simulink model "Gesamtsystem_Prototyp25_01_3"  (R2021b)
settings: Solver=FixedStepDiscrete  StartTime=0.0  StopTime=Inf  RelTol=1e-3  EnableMultiTasking=on
undefined symbols (not defined in the file): Down, GPTRIP1SEL, GPTRIP2SEL, magnitude, TZ1, TZ2, Up
libraries: c2837xDlib x18, hdlsllib x10, simulink x5, c2802xlib x5, c280xlib x3, dspsigops x3, commsequence2 x2, idelinklib_common x2, mcbcontrolslib x2, c2000lib x1, dspstat3 x1
(part 1 of 3)
settings Model: SimulationMode=external  ExtModeTrigDuration=8  Creator=The MathWorks, Inc.  LastModifiedBy=richa
settings SolverCC: AlgebraicLoopSolver=TrustRegion
settings OptimizationCC: DefaultUnderspecifiedDataType=single  EnhancedBackFolding=on  PassReuseOutputArgsAs=Individual arguments  MaxStackSize=1024  OptimizeBlockOrder=speed  DifferentSizesBufferReuse=on  OptimizationCustomize=off  DenormalBehavior=FlushToZero  EfficientTunableParamExpr=on
settings DebuggingCC: MultiTaskRateTransMsg=warning  ParameterTunabilityLossMsg=error  SFMachineParentedDataDiag=warning
settings HardwareCC: ProdBitPerChar=16  ProdBitPerInt=16  ProdBitPerPointer=32  ProdBitPerSizeT=32  ProdBitPerPtrDiffT=32  ProdLargestAtomicInteger=Integer  ProdLargestAtomicFloat=None  ProdWordSize=16  ProdLongLongMode=on  ProdHWDeviceType=Texas Instruments->C2000
settings SFSimCC: SimCustomSourceCode="#include \"i2c_reset.c\""  SimCustomHeaderCode="#include \"i2c_reset.h\""  MATLABDynamicMemAlloc=off
settings RTWCC: Description=Embedded Coder  SystemTargetFile=ert.tlc  HardwareBoard=TI Delfino F28379D LaunchPad  TemplateMakefile=ert_default_tmf  GenerateReport=on  RTWUseSimCustomCode=on  CustomSourceCode="#include \"i2c_reset.c\""  CustomHeaderCode="#include \"i2c_reset.h\""  Toolchain=Texas Instruments Code Composer Studio (C2000)
settings CodeAppCC: ForceParamTrailComments=on  IgnoreCustomStorageClasses=off  OperatorAnnotations=on  SimulinkDataObjDesc=on  SFDataObjDesc=on  InsertBlockDesc=on
settings ERTTargetCC: CodeReplacementLibrary=TI C28x  SupportContinuousTime=on  ExtMode=on  ExtModeTransport=4  ExtModeStaticAlloc=on  ExtModeStaticAllocSize=10000  ExtModeMexFile=ext_xcp  ExtModeMexArgs=1 7 5000000  ExtModeIntrfLevel=Level2 - Open

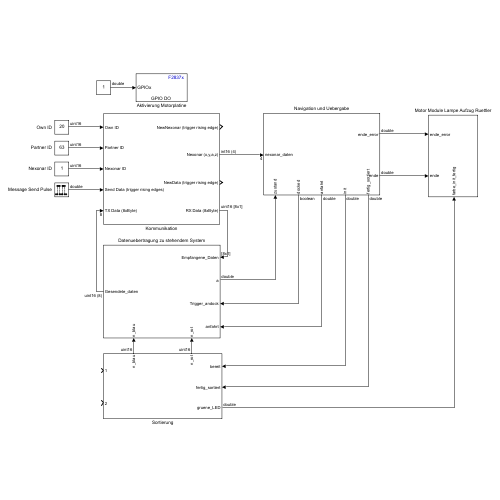
[thumbnail: Simulink's stored preview of the top-level diagram]
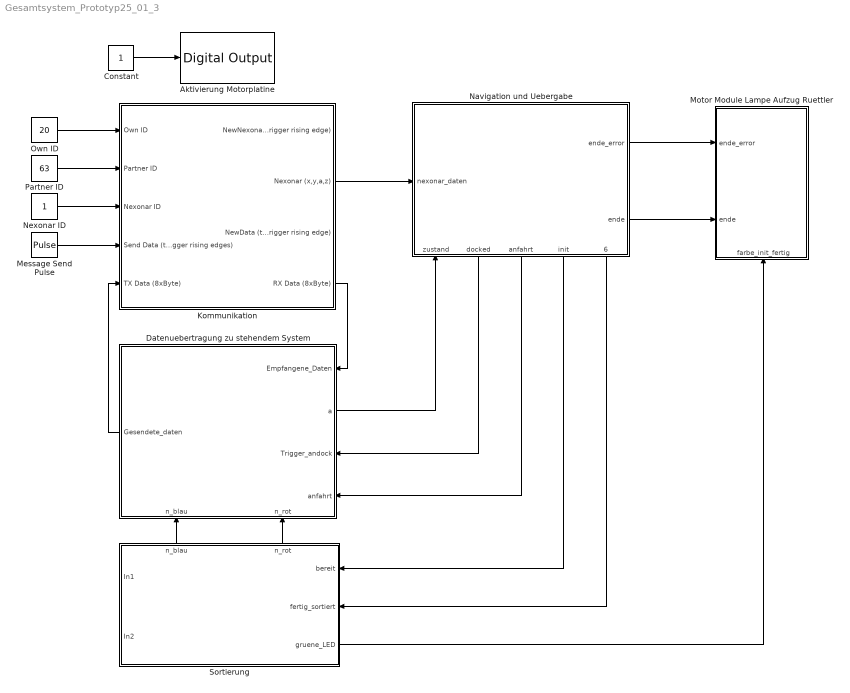
== system Gesamtsystem_Prototyp25_01_3 ==
  Aktivierung Motorplatine : c2837xDlib/Digital Output  GPIO_Number=GPIO48~GPIO55  GPIO_Bit0=off  GPIO_BIT0_Toggle=on  GPIO_Bit1=off  GPIO_BIT1_Toggle=off  GPIO_Bit2=off  GPIO_BIT2_Toggle=off  GPIO_Bit3=off  GPIO_BIT3_Toggle=off  GPIO_Bit4=on  GPIO_BIT4_Toggle=on  GPIO_Bit5=off  GPIO_BIT5_Toggle=off  GPIO_Bit6=off  GPIO_BIT6_Toggle=off  GPIO_Bit7=off  GPIO_BIT7_Toggle=off
      settings: SourceProductBaseCode=TIC2000
  Constant : Constant
  Datenuebertragung zu stehendem System : Subsystem
      settings: PortSchema="{\"entries\":[{\"content\":{\"sides\":[{\"content\":{\"connectorIds\":[\"Out2\"]},\"type\":\"ConnectorPlacement.EquallySpacedRectSide\",\"uuid\":\"280a4ad7-2b89-47a7-b582-5b9e1aa8e579\"},{\"content\":{\"connectorIds\":[\"In3\",\"Out1\",\"In4\",\"In5\"],\"side\":\"RIGHT\"},\"type\":\"ConnectorPlacement.EquallySpacedRectSide\",\"uuid\":\"026a8d37-e820-494f-976a-b1ab356a46bf\"},{\"content\":{\"connectorIds\":[],\"side\":\"TOP\"},\"type\":\"ConnectorPlacement.EquallySpacedRectSide\",\"uuid\":\"c41355c1-e8ef-4a5b-90ea-c5b98acbcd23\"},{\"content\":{\"connectorIds\":[\"In1\",\"In2\"],\"side\":\"BOTTOM\"},\"type\":\"ConnectorPlacement.EquallySpacedRectSide\",\"uuid\":\"0f189695-a2e5-45de-b8d0-0b48a4f2d2d4\"}]},\"type\":\"ConnectorPlacement.EquallySpacedConnector\",\"uuid\":\"44cb629b-e0dd-4ad8-b455-e727a6a25bea\"}],\"packageUris\":[\"http://schema.mathworks.com/mf0/Connector/R2020b\"],\"version\":\"1.0\"}"
  Kommunikation : Subsystem
  Message Send Pulse : DiscretePulseGenerator  SampleTime=0.25
  Motor Module Lampe Aufzug Ruettler : Subsystem
      settings: PortSchema="{\"entries\":[{\"content\":{\"sides\":[{\"content\":{\"connectorIds\":[\"In1\",\"In2\"]},\"type\":\"ConnectorPlacement.EquallySpacedRectSide\",\"uuid\":\"9123dc57-6e13-4d06-96d5-694d4c57ade7\"},{\"content\":{\"connectorIds\":[],\"side\":\"RIGHT\"},\"type\":\"ConnectorPlacement.EquallySpacedRectSide\",\"uuid\":\"65464e42-9400-426f-8ced-3069c16bd5e7\"},{\"content\":{\"connectorIds\":[],\"side\":\"TOP\"},\"type\":\"ConnectorPlacement.EquallySpacedRectSide\",\"uuid\":\"b48c1543-2088-461c-846d-d08a40b96f4c\"},{\"content\":{\"connectorIds\":[\"In3\"],\"side\":\"BOTTOM\"},\"type\":\"ConnectorPlacement.EquallySpacedRectSide\",\"uuid\":\"aa8ff81a-6422-494d-aeab-2069a4a6b426\"}]},\"type\":\"ConnectorPlacement.EquallySpacedConnector\",\"uuid\":\"98b07be5-fb16-44db-b7cc-951c09166bfd\"}],\"packageUris\":[\"http://schema.mathworks.com/mf0/Connector/R2020b\"],\"version\":\"1.0\"}"
  Navigation und Uebergabe : Subsystem
      settings: PortSchema="{\"entries\":[{\"content\":{\"sides\":[{\"content\":{\"connectorIds\":[\"In1\"]},\"type\":\"ConnectorPlacement.EquallySpacedRectSide\",\"uuid\":\"dfc964e5-dd2b-4b2e-9c3a-c7814fa8e123\"},{\"content\":{\"connectorIds\":[\"Out1\",\"Out2\"],\"side\":\"RIGHT\"},\"type\":\"ConnectorPlacement.EquallySpacedRectSide\",\"uuid\":\"39fc11e7-81f7-4c6b-bd33-df7afb59ff58\"},{\"content\":{\"connectorIds\":[],\"side\":\"TOP\"},\"type\":\"ConnectorPlacement.EquallySpacedRectSide\",\"uuid\":\"36c4a621-1407-48e7-9ea9-d5e57de15753\"},{\"content\":{\"connectorIds\":[\"In2\",\"Out3\",\"Out4\",\"Out5\",\"Out6\"],\"side\":\"BOTTOM\"},\"type\":\"ConnectorPlacement.EquallySpacedRectSide\",\"uuid\":\"43cd8641-88b7-45a0-ae78-0764539c8380\"}]},\"type\":\"ConnectorPlacement.EquallySpacedConnector\",\"uuid\":\"ac412e3d-8275-4bb9-9e3f-1b0a94176768\"}],\"packageUris\":[\"http://schema.mathworks.com/mf0/Connector/R2020b\"],\"version\":\"1.0\"}"
  Nexonar ID : Constant  OutDataTypeStr=uint16
  Own ID : Constant  Value=20  OutDataTypeStr=uint16
  Partner ID : Constant  Value=63  OutDataTypeStr=uint16
  Sortierung : Subsystem
      settings: PortSchema="{\"entries\":[{\"content\":{\"sides\":[{\"content\":{\"connectorIds\":[\"In1\",\"In2\"]},\"type\":\"ConnectorPlacement.EquallySpacedRectSide\",\"uuid\":\"ab30f80d-c1d3-46e0-874b-ff067c3feed5\"},{\"content\":{\"connectorIds\":[\"In3\",\"In4\",\"Out1\"],\"side\":\"RIGHT\"},\"type\":\"ConnectorPlacement.EquallySpacedRectSide\",\"uuid\":\"516d9c97-20f8-430b-a7d3-5b8718eca889\"},{\"content\":{\"connectorIds\":[\"Out2\",\"Out3\"],\"side\":\"TOP\"},\"type\":\"ConnectorPlacement.EquallySpacedRectSide\",\"uuid\":\"26f872a1-b740-4d7b-a87d-ca1faf51abaa\"},{\"content\":{\"connectorIds\":[],\"side\":\"BOTTOM\"},\"type\":\"ConnectorPlacement.EquallySpacedRectSide\",\"uuid\":\"97241500-f762-4060-9f54-e0d97a9e1284\"}]},\"type\":\"ConnectorPlacement.EquallySpacedConnector\",\"uuid\":\"cf514a40-a14e-4820-a098-62891cb48e81\"}],\"packageUris\":[\"http://schema.mathworks.com/mf0/Connector/R2020b\"],\"version\":\"1.0\"}"
  wires:
  Constant/1 -> Aktivierung Motorplatine/1
  Partner ID/1 -> Kommunikation/2(Partner ID)
  Own ID/1 -> Kommunikation/1(Own ID)
  Nexonar ID/1 -> Kommunikation/3(Nexonar ID)
  Message Send Pulse/1 -> Kommunikation/4(Send Data (trigger rising edges))
  Kommunikation/2(Nexonar (x,y,a,z)) -> Navigation und Uebergabe/1(nexonar_daten)
  Navigation und Uebergabe/2(ende) -> Motor Module Lampe Aufzug Ruettler/2(ende)
  Kommunikation/4(RX Data (8xByte)) -> Datenuebertragung zu stehendem System/3(Empfangene_Daten)
  Datenuebertragung zu stehendem System/2(Gesendete_daten) -> Kommunikation/5(TX Data (8xByte))
  Datenuebertragung zu stehendem System/1(a) -> Navigation und Uebergabe/2(zustand)
  Sortierung/2(n_blau) -> Datenuebertragung zu stehendem System/1(n_blau)
  Sortierung/3(n_rot) -> Datenuebertragung zu stehendem System/2(n_rot)
  Navigation und Uebergabe/4(anfahrt) -> Datenuebertragung zu stehendem System/5(anfahrt)
  Navigation und Uebergabe/5(init) -> Sortierung/3(bereit)
  Sortierung/1(gruene_LED) -> Motor Module Lampe Aufzug Ruettler/3(farbe_init_fertig)
  Navigation und Uebergabe/3(docked) -> Datenuebertragung zu stehendem System/4(Trigger_andock)
  Navigation und Uebergabe/1(ende_error) -> Motor Module Lampe Aufzug Ruettler/1(ende_error)
  Navigation und Uebergabe/6(fertig_sortiert) -> Sortierung/4(fertig_sortiert)

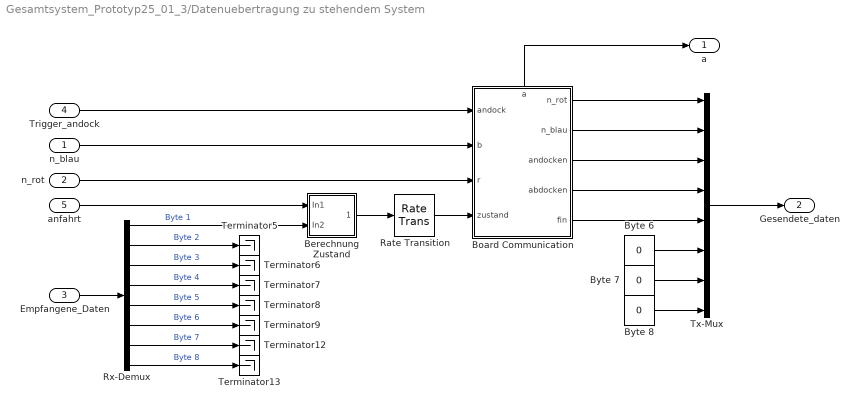
== system Gesamtsystem_Prototyp25_01_3/Datenuebertragung zu stehendem System ==
  n_blau : Inport
  n_rot : Inport  Port=2
  Empfangene_Daten : Inport  Port=3
  Trigger_andock : Inport  Port=4
  anfahrt : Inport  Port=5
  Berechnung Zustand : Subsystem
  Board Communication : Stateflow chart  TreatAsAtomicUnit=on
      settings: PortSchema="{\"entries\":[{\"content\":{\"sides\":[{\"content\":{\"connectorIds\":[\"In4\",\"In1\",\"In2\",\"In3\"]},\"type\":\"ConnectorPlacement.EquallySpacedRectSide\",\"uuid\":\"faa8cb3d-0fdf-435a-9df5-bd02dffb58bc\"},{\"content\":{\"connectorIds\":[\"Out1\",\"Out5\",\"Out3\",\"Out4\",\"Out6\"],\"side\":\"RIGHT\"},\"type\":\"ConnectorPlacement.EquallySpacedRectSide\",\"uuid\":\"4764847e-6149-4239-b002-0e5a6e767122\"},{\"content\":{\"connectorIds\":[\"Out2\"],\"side\":\"TOP\"},\"type\":\"ConnectorPlacement.EquallySpacedRectSide\",\"uuid\":\"2cc71a59-6d23-41ec-a2d6-96294ff626b2\"}]},\"type\":\"ConnectorPlacement.EquallySpacedConnector\",\"uuid\":\"aa42c799-a033-4d4d-b66c-54ab2872aaa8\"}],\"packageUris\":[\"http://schema.mathworks.com/mf0/Connector/R2020b\"],\"version\":\"1.0\"}"
  Byte 6 : Constant  Value=0  OutDataTypeStr=uint16
  Byte 7 : Constant  Value=0  OutDataTypeStr=uint16
  Byte 8 : Constant  Value=0  OutDataTypeStr=uint16
  Rate Transition : RateTransition  OutPortSampleTime=0.2
  Rx-Demux : Demux  Outputs=8
  Terminator{5..9,12..13} (7 alike) : Terminator
  Tx-Mux : Mux  Inputs=8
  a : Outport
  Gesendete_daten : Outport  Port=2
  wires:
  Rx-Demux/3 -> Terminator6/1  "Byte 3"
  Board Communication/3(andocken) -> Tx-Mux/3
  Rx-Demux/1 -> Berechnung Zustand/2(In2)  "Byte 1"
  Rx-Demux/6 -> Terminator9/1  "Byte 6"
  Berechnung Zustand/1(zustand) -> Rate Transition/1
  Board Communication/5(n_blau) -> Tx-Mux/2
  Rx-Demux/4 -> Terminator7/1  "Byte 4"
  Byte 8/1 -> Tx-Mux/8
  Byte 7/1 -> Tx-Mux/7
  Rx-Demux/5 -> Terminator8/1  "Byte 5"
  Rx-Demux/8 -> Terminator13/1  "Byte 8"
  Byte 6/1 -> Tx-Mux/6
  Rx-Demux/7 -> Terminator12/1  "Byte 7"
  Board Communication/6(fin) -> Tx-Mux/5
  Tx-Mux/1 -> Gesendete_daten/1
  Board Communication/4(abdocken) -> Tx-Mux/4
  Rx-Demux/2 -> Terminator5/1  "Byte 2"
  Board Communication/1(n_rot) -> Tx-Mux/1
  Empfangene_Daten/1 -> Rx-Demux/1
  n_rot/1 -> Board Communication/2(r)
  Trigger_andock/1 -> Board Communication/4(andock)
  n_blau/1 -> Board Communication/1(b)
  Board Communication/2(a) -> a/1
  Rate Transition/1 -> Board Communication/3(zustand)
  anfahrt/1 -> Berechnung Zustand/1(In1)

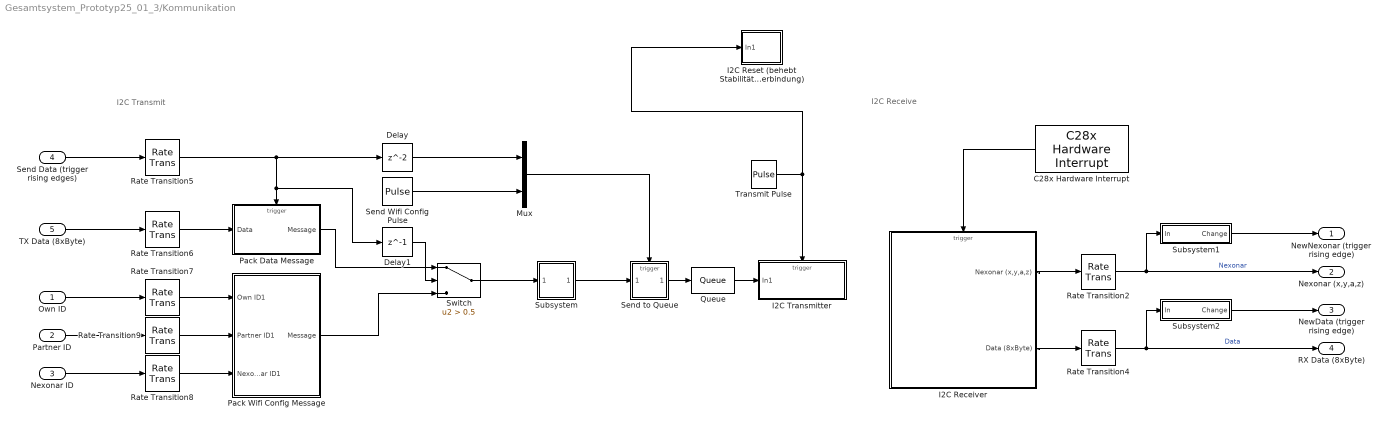
== system Gesamtsystem_Prototyp25_01_3/Kommunikation ==
  note: I2C Receive
  note: I2C Transmit
  Own ID : Inport
  Partner ID : Inport  Port=2
  Nexonar ID : Inport  Port=3
  Send Data (trigger rising edges) : Inport  Port=4
  TX Data (8xByte) : Inport  Port=5
  C28x Hardware Interrupt : c2000lib/Scheduling/C28x Hardware Interrupt  irqnumbers=8  pienumbers=2  irqpriorities=30  irqpreempts=0  showinput=off  dspchiptype=C280X
      settings: SourceProductBaseCode=TIC2000
  Delay : Delay
  Delay1 : Delay  DelayLength=1
  I2C Receiver : Subsystem  TreatAsAtomicUnit=on
  I2C Reset (behebt Stabilitätsprobleme der I2C-Verbindung) : Subsystem
  I2C Transmitter : Subsystem
  Mux : Mux  Inputs=2
  Pack Data Message : Subsystem
  Pack Wifi Config Message : Subsystem
  Queue : Queue  InputPortMessageModes=m  OutputPortMessageModes=m  OverwriteOldest=on  Capacity=16
  Rate Transition2 : RateTransition  Deterministic=off  OutPortSampleTime=0.01
  Rate Transition4 : RateTransition  Deterministic=off  OutPortSampleTime=0.01
  Rate Transition{5..9} (5 alike) : RateTransition  Deterministic=off  OutPortSampleTimeOpt=Inherit  OutPortSampleTime=0.01
  Send Wifi Config Pulse : DiscretePulseGenerator  Period=10  PhaseDelay=30  SampleTime=0.01
  Send to Queue : Subsystem
  Subsystem : Subsystem
  Subsystem1 : Subsystem
  Subsystem2 : Subsystem
  Switch : Switch  Criteria=u2 > Threshold  Threshold=0.5
  Transmit Pulse : DiscretePulseGenerator  Period=100  PulseWidth=5  SampleTime=0.001
  NewNexonar (trigger rising edge) : Outport
  Nexonar (x,y,a,z) : Outport  Port=2
  NewData (trigger rising edge) : Outport  Port=3
  RX Data (8xByte) : Outport  Port=4
  wires:
  I2C Receiver/1(Nexonar (x,y,a,z)) -> Rate Transition2/1
  Rate Transition2/1 -> Subsystem1/1(In), Nexonar (x,y,a,z)/1  "Nexonar"
  C28x Hardware Interrupt/1 -> I2C Receiver/Trigger
  I2C Receiver/2(Data (8xByte)) -> Rate Transition4/1
  Rate Transition4/1 -> Subsystem2/1(In), RX Data (8xByte)/1  "Data"
  Queue/1 -> I2C Transmitter/1(In1)
  Send to Queue/1(Out1) -> Queue/1
  Pack Data Message/1(Message) -> Switch/1
  Pack Wifi Config Message/1(Message) -> Switch/3
  Delay/1 -> Mux/1
  Mux/1 -> Send to Queue/Trigger
  Delay1/1 -> Switch/2
  Send Data (trigger rising edges)/1 -> Rate Transition5/1
  TX Data (8xByte)/1 -> Rate Transition6/1
  Rate Transition6/1 -> Pack Data Message/1(Data)
  Rate Transition9/1 -> Pack Wifi Config Message/2(Partner ID1)
  Partner ID/1 -> Rate Transition9/1
  Own ID/1 -> Rate Transition7/1
  Rate Transition7/1 -> Pack Wifi Config Message/1(Own ID1)
  Nexonar ID/1 -> Rate Transition8/1
  Rate Transition8/1 -> Pack Wifi Config Message/3(Nexonar ID1)
  Rate Transition5/1 -> Delay/1, Pack Data Message/Trigger, Delay1/1
  Switch/1 -> Subsystem/1(In1)
  Subsystem/1(Out1) -> Send to Queue/1(In1)
  Send Wifi Config Pulse/1 -> Mux/2
  Subsystem1/1(Change) -> NewNexonar (trigger rising edge)/1
  Subsystem2/1(Change) -> NewData (trigger rising edge)/1
  Transmit Pulse/1 -> I2C Reset (behebt Stabilitätsprobleme der I2C-Verbindung)/1(In1), I2C Transmitter/Trigger

== system Gesamtsystem_Prototyp25_01_3/Motor Module Lampe Aufzug Ruettler ==
  ende_error : Inport
  ende : Inport  Port=2
  farbe_init_fertig : Inport  Port=3
  Aufzug : c2837xDlib/Digital Output  GPIO_Number=GPIO104~GPIO111  GPIO_Bit0=off  GPIO_BIT0_Toggle=off  GPIO_Bit1=off  GPIO_BIT1_Toggle=off  GPIO_Bit2=off  GPIO_BIT2_Toggle=off  GPIO_Bit3=off  GPIO_BIT3_Toggle=off  GPIO_Bit4=off  GPIO_BIT4_Toggle=off  GPIO_Bit5=off  GPIO_BIT5_Toggle=off  GPIO_Bit6=off  GPIO_BIT6_Toggle=off  GPIO_Bit7=on  GPIO_BIT7_Toggle=off
      settings: SourceProductBaseCode=TIC2000
  Endlicht : c2837xDlib/Digital Output  GPIO_Number=GPIO64~GPIO71  GPIO_Bit0=off  GPIO_BIT0_Toggle=off  GPIO_Bit1=off  GPIO_BIT1_Toggle=off  GPIO_Bit2=off  GPIO_BIT2_Toggle=off  GPIO_Bit3=on  GPIO_BIT3_Toggle=off  GPIO_Bit4=off  GPIO_BIT4_Toggle=off  GPIO_Bit5=off  GPIO_BIT5_Toggle=off  GPIO_Bit6=off  GPIO_BIT6_Toggle=off  GPIO_Bit7=off  GPIO_BIT7_Toggle=off
      settings: SourceProductBaseCode=TIC2000
  Inverter : Subsystem
  Logical Operator : Logic  AllPortsSameDT=off  OutDataTypeStr=boolean
  Logical Operator1 : Logic  Operator=OR  AllPortsSameDT=off  OutDataTypeStr=boolean
  wires:
  Logical Operator1/1 -> Logical Operator/2, Inverter/1(ende)
  Inverter/1(ende_nicht) -> Aufzug/1
  Logical Operator/1 -> Endlicht/1
  farbe_init_fertig/1 -> Logical Operator/1
  ende_error/1 -> Logical Operator1/2
  ende/1 -> Logical Operator1/1

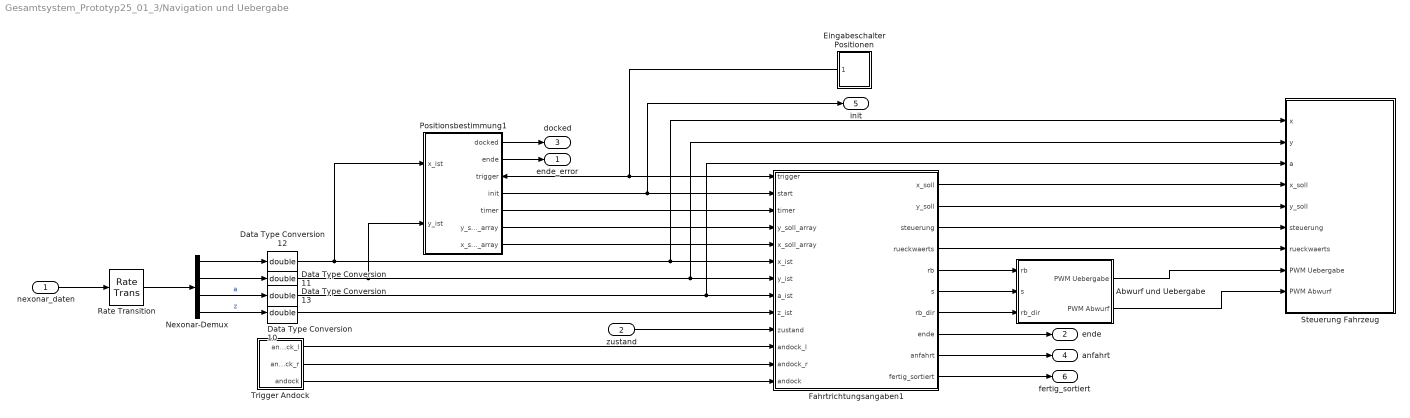
== system Gesamtsystem_Prototyp25_01_3/Navigation und Uebergabe ==
  nexonar_daten : Inport
  zustand : Inport  Port=2
  Abwurf und Uebergabe : Subsystem
  Data Type Conversion{10..13} (4 alike) : DataTypeConversion  OutDataTypeStr=double
  Eingabeschalter Positionen : Subsystem
      settings: PortSchema="{\"entries\":[{\"content\":{\"sides\":[{\"content\":{\"connectorIds\":[\"Out1\"]},\"type\":\"ConnectorPlacement.EquallySpacedRectSide\",\"uuid\":\"1d6011d2-9ec8-4188-a4ee-29e3da0b2ada\"},{\"content\":{\"connectorIds\":[],\"side\":\"RIGHT\"},\"type\":\"ConnectorPlacement.EquallySpacedRectSide\",\"uuid\":\"dfaa9298-af69-413c-bedd-37923d151273\"},{\"content\":{\"connectorIds\":[],\"side\":\"TOP\"},\"type\":\"ConnectorPlacement.EquallySpacedRectSide\",\"uuid\":\"6f8c24f7-9703-40ab-ade9-63e7bbae06cc\"},{\"content\":{\"connectorIds\":[],\"side\":\"BOTTOM\"},\"type\":\"ConnectorPlacement.EquallySpacedRectSide\",\"uuid\":\"8969ef2b-e70c-4a01-a0ba-7054fd594c62\"}]},\"type\":\"ConnectorPlacement.EquallySpacedConnector\",\"uuid\":\"29177e89-d61b-4a13-8f11-081f64dd03c8\"}],\"packageUris\":[\"http://schema.mathworks.com/mf0/Connector/R2020b\"],\"version\":\"1.0\"}"
  Fahrtrichtungsangaben1 : Stateflow chart  TreatAsAtomicUnit=on
      settings: PortSchema="{\"entries\":[{\"content\":{\"sides\":[{\"content\":{\"connectorIds\":[\"In1\",\"In4\",\"In2\",\"In9\",\"In10\",\"In5\",\"In6\",\"In7\",\"In8\",\"In11\",\"In12\",\"In13\",\"In3\"]},\"type\":\"ConnectorPlacement.EquallySpacedRectSide\",\"uuid\":\"a52a4362-e7c3-41ca-812a-cc890816dcdf\"},{\"content\":{\"connectorIds\":[\"Out5\",\"Out7\",\"Out6\",\"Out4\",\"Out3\",\"Out2\",\"Out10\",\"Out1\",\"Out8\",\"Out9\"],\"side\":\"RIGHT\"},\"type\":\"ConnectorPlacement.EquallySpacedRectSide\",\"uuid\":\"87550de2-1a7b-4795-9189-02306bbe50b1\"},{\"content\":{\"connectorIds\":[],\"side\":\"TOP\"},\"type\":\"ConnectorPlacement.EquallySpacedRectSide\",\"uuid\":\"5e6e6b57-2edc-428f-ba9f-6f661fb7c808\"},{\"content\":{\"connectorIds\":[],\"side\":\"BOTTOM\"},\"type\":\"ConnectorPlacement.EquallySpacedRectSide\",\"uuid\":\"36c63001-0682-4bf8-b83c-9f123a4632ed\"}]},\"type\":\"ConnectorPlacement.EquallySpacedConnector\",\"uuid\":\"d6e0e4fe-fc35-4bad-a417-b8cbd6698281\"}],\"packageUris\":[\"http://schema.mathworks.com/mf0/Connector/R2020b\"],\"version\":\"1.0\"}"
  Nexonar-Demux : Demux
  Positionsbestimmung1 : Stateflow chart  TreatAsAtomicUnit=on
      settings: PortSchema="{\"entries\":[{\"content\":{\"sides\":[{\"content\":{\"connectorIds\":[\"In2\",\"In3\"]},\"type\":\"ConnectorPlacement.EquallySpacedRectSide\",\"uuid\":\"5fe3459d-aa84-4ddc-8aa7-ba930fd4ad02\"},{\"content\":{\"connectorIds\":[\"Out1\",\"Out6\",\"In1\",\"Out4\",\"Out3\",\"Out5\",\"Out2\"],\"side\":\"RIGHT\"},\"type\":\"ConnectorPlacement.EquallySpacedRectSide\",\"uuid\":\"d03efab7-855f-477c-bf79-639f3e2a0475\"},{\"content\":{\"connectorIds\":[],\"side\":\"TOP\"},\"type\":\"ConnectorPlacement.EquallySpacedRectSide\",\"uuid\":\"85444a67-c2c0-4585-ab9c-7839844ad5c4\"}]},\"type\":\"ConnectorPlacement.EquallySpacedConnector\",\"uuid\":\"5918b77a-04f6-4ee4-be1c-1d10f015dccb\"}],\"packageUris\":[\"http://schema.mathworks.com/mf0/Connector/R2020b\"],\"version\":\"1.0\"}"
  Rate Transition : RateTransition  OutPortSampleTime=0.1
  Steuerung Fahrzeug : Subsystem
  Trigger Andock : Subsystem
  ende_error : Outport
  ende : Outport  Port=2
  docked : Outport  Port=3
  anfahrt : Outport  Port=4
  init : Outport  Port=5
  fertig_sortiert : Outport  Port=6
  wires:
  Abwurf und Uebergabe/2(PWM Abwurf) -> Steuerung Fahrzeug/9(PWM Abwurf)
  Abwurf und Uebergabe/1(PWM Uebergabe) -> Steuerung Fahrzeug/8(PWM Uebergabe)
  Fahrtrichtungsangaben1/5(x_soll) -> Steuerung Fahrzeug/4(x_soll)
  Fahrtrichtungsangaben1/2(s) -> Abwurf und Uebergabe/2(s)
  Nexonar-Demux/3 -> Data Type Conversion13/1  "a"
  Nexonar-Demux/4 -> Data Type Conversion10/1  "z"
  Data Type Conversion10/1 -> Fahrtrichtungsangaben1/8(z_ist)
  Fahrtrichtungsangaben1/6(steuerung) -> Steuerung Fahrzeug/6(steuerung)
  Fahrtrichtungsangaben1/7(y_soll) -> Steuerung Fahrzeug/5(y_soll)
  Nexonar-Demux/2 -> Data Type Conversion11/1
  Fahrtrichtungsangaben1/1(ende) -> ende/1
  Nexonar-Demux/1 -> Data Type Conversion12/1
  Data Type Conversion13/1 -> Steuerung Fahrzeug/3(a), Fahrtrichtungsangaben1/7(a_ist)
  Fahrtrichtungsangaben1/4(rueckwaerts) -> Steuerung Fahrzeug/7(rueckwaerts)
  Fahrtrichtungsangaben1/3(rb) -> Abwurf und Uebergabe/1(rb)
  nexonar_daten/1 -> Rate Transition/1
  Rate Transition/1 -> Nexonar-Demux/1
  zustand/1 -> Fahrtrichtungsangaben1/11(zustand)
  Trigger Andock/1(andock_l) -> Fahrtrichtungsangaben1/12(andock_l)
  Trigger Andock/2(andock_r) -> Fahrtrichtungsangaben1/13(andock_r)
  Trigger Andock/3(andock) -> Fahrtrichtungsangaben1/3(andock)
  Data Type Conversion11/1 -> Positionsbestimmung1/3(y_ist), Steuerung Fahrzeug/2(y), Fahrtrichtungsangaben1/6(y_ist)
  Data Type Conversion12/1 -> Positionsbestimmung1/2(x_ist), Steuerung Fahrzeug/1(x), Fahrtrichtungsangaben1/5(x_ist)
  Positionsbestimmung1/2(x_soll_array) -> Fahrtrichtungsangaben1/10(x_soll_array)
  Positionsbestimmung1/4(init) -> init/1, Fahrtrichtungsangaben1/4(start)
  Positionsbestimmung1/5(y_soll_array) -> Fahrtrichtungsangaben1/9(y_soll_array)
  Eingabeschalter Positionen/1(trigger) -> Positionsbestimmung1/1(trigger), Fahrtrichtungsangaben1/1(trigger)
  Fahrtrichtungsangaben1/8(anfahrt) -> anfahrt/1
  Positionsbestimmung1/3(timer) -> Fahrtrichtungsangaben1/2(timer)
  Fahrtrichtungsangaben1/10(rb_dir) -> Abwurf und Uebergabe/3(rb_dir)
  Positionsbestimmung1/1(docked) -> docked/1
  Positionsbestimmung1/6(ende) -> ende_error/1
  Fahrtrichtungsangaben1/9(fertig_sortiert) -> fertig_sortiert/1

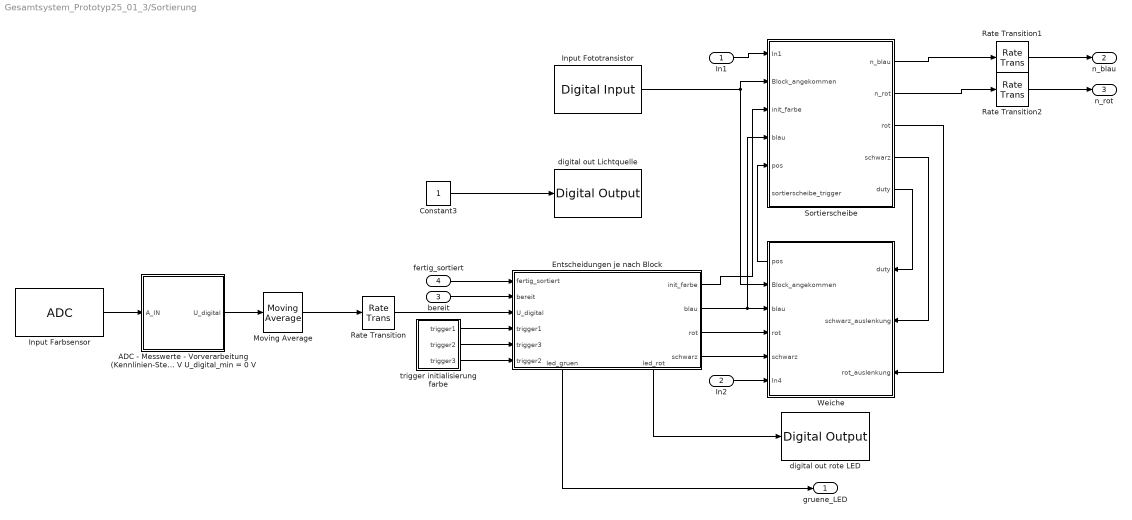
== system Gesamtsystem_Prototyp25_01_3/Sortierung ==
  In1 : Inport
  In2 : Inport  Port=2
  bereit : Inport  Port=3
  fertig_sortiert : Inport  Port=4
  ADC - Messwerte - Vorverarbeitung (Kennlinien-Steigung und Offset-Kompensation) U_digital = (ADC_in - Offset) * 4.505 V / 4096 mit U_digital_max = 4.505 V U_digital_min = 0 V : Subsystem
  Constant3 : Constant
  Entscheidungen je nach Block : Stateflow chart  TreatAsAtomicUnit=on
      settings: PortSchema="{\"entries\":[{\"content\":{\"sides\":[{\"content\":{\"connectorIds\":[\"In1\",\"In5\",\"In6\",\"In2\",\"In3\",\"In4\"]},\"type\":\"ConnectorPlacement.EquallySpacedRectSide\",\"uuid\":\"f09b8754-b634-4b2b-b5bd-16eb62568de2\"},{\"content\":{\"connectorIds\":[\"Out6\",\"Out5\",\"Out3\",\"Out4\"],\"side\":\"RIGHT\"},\"type\":\"ConnectorPlacement.EquallySpacedRectSide\",\"uuid\":\"354cc761-a49e-425d-8c72-e7db509e3167\"},{\"content\":{\"connectorIds\":[],\"side\":\"TOP\"},\"type\":\"ConnectorPlacement.EquallySpacedRectSide\",\"uuid\":\"bd0f8b9d-16c9-4d23-ab04-a69da24b10b6\"},{\"content\":{\"connectorIds\":[\"Out1\",\"Out2\"],\"side\":\"BOTTOM\"},\"type\":\"ConnectorPlacement.EquallySpacedRectSide\",\"uuid\":\"af3469b1-ebbb-44bc-bbc8-b4348fb1f080\"}]},\"type\":\"ConnectorPlacement.EquallySpacedConnector\",\"uuid\":\"f6f99529-e417-4cea-b92d-fd20e5779b1a\"}],\"packageUris\":[\"http://schema.mathworks.com/mf0/Connector/R2020b\"],\"version\":\"1.0\"}"
  Input Farbsensor : c2802xlib/ADC  blkParamProc=C2000_Type4  ADCModule=A  samplingMode=Single sample mode  ADCResolution=12-bit (Single-ended input)  useSOC1=SOC14  useSOC2=SOC0_SOC1  SOCAcquisitionWindow=15  SOCTriggerSource=Software  SOCInterruptTrigger=No ADCINT  Ts=0.001  dType=uint16  postInterrupt=off  interruptSel=ADCINT1  ADCINTContinuous=on  endma=off  chdma=1  conv1=ADCINA0  conv2=ADCINA0 and ADCINB0  conv1_Type4=ADCIN14  conv2_Type4=ADCIN0 and ADCIN1
  Input Fototransistor : c2837xDlib/Digital Input  GPIO_Number=GPIO0~GPIO7  GPIO_Bit0=off  GPIO_Bit1=off  GPIO_Bit2=on  GPIO_Bit3=off  GPIO_Bit4=off  GPIO_Bit5=off  GPIO_Bit6=off  GPIO_Bit7=off  sampleTime=0.1  dataType=auto  GPIO_Bit0_Qualification=Sync to SYSCLKOUT  GPIO_Bit1_Qualification=Sync to SYSCLKOUT  GPIO_Bit2_Qualification=Sync to SYSCLKOUT  GPIO_Bit3_Qualification=Sync to SYSCLKOUT  GPIO_Bit4_Qualification=Sync to SYSCLKOUT  GPIO_Bit5_Qualification=Sync to SYSCLKOUT  GPIO_Bit6_Qualification=Sync to SYSCLKOUT  GPIO_Bit7_Qualification=Sync to SYSCLKOUT  Qualification_Period=-1
      settings: SourceProductBaseCode=TIC2000
  Moving Average : dspstat3/Moving Average  Method=Sliding window  ForgettingFactorPort=off  SpecifyWindowLength=on  WindowLength=50  ForgettingFactor=0.9  SimulateUsing=Code generation
  Rate Transition : RateTransition  OutPortSampleTime=0.1
  Rate Transition1 : RateTransition  OutPortSampleTime=0.2
  Rate Transition2 : RateTransition  OutPortSampleTime=0.2
  Sortierscheibe : Subsystem
  Weiche : Subsystem
      settings: PortSchema="{\"entries\":[{\"content\":{\"sides\":[{\"content\":{\"connectorIds\":[\"Out1\",\"In1\",\"In2\",\"In3\",\"In4\",\"In5\"]},\"type\":\"ConnectorPlacement.EquallySpacedRectSide\",\"uuid\":\"280a4ad7-2b89-47a7-b582-5b9e1aa8e579\"},{\"content\":{\"connectorIds\":[\"In6\",\"In7\",\"In8\"],\"side\":\"RIGHT\"},\"type\":\"ConnectorPlacement.EquallySpacedRectSide\",\"uuid\":\"026a8d37-e820-494f-976a-b1ab356a46bf\"},{\"content\":{\"connectorIds\":[],\"side\":\"TOP\"},\"type\":\"ConnectorPlacement.EquallySpacedRectSide\",\"uuid\":\"c41355c1-e8ef-4a5b-90ea-c5b98acbcd23\"}]},\"type\":\"ConnectorPlacement.EquallySpacedConnector\",\"uuid\":\"44cb629b-e0dd-4ad8-b455-e727a6a25bea\"}],\"packageUris\":[\"http://schema.mathworks.com/mf0/Connector/R2020b\"],\"version\":\"1.0\"}"
  digital out Lichtquelle : c2837xDlib/Digital Output  GPIO_Number=GPIO32~GPIO39  GPIO_Bit0=on  GPIO_BIT0_Toggle=off  GPIO_Bit1=off  GPIO_BIT1_Toggle=off  GPIO_Bit2=off  GPIO_BIT2_Toggle=off  GPIO_Bit3=off  GPIO_BIT3_Toggle=off  GPIO_Bit4=off  GPIO_BIT4_Toggle=on  GPIO_Bit5=off  GPIO_BIT5_Toggle=off  GPIO_Bit6=off  GPIO_BIT6_Toggle=off  GPIO_Bit7=off  GPIO_BIT7_Toggle=off
      settings: SourceProductBaseCode=TIC2000
  digital out rote LED : c2837xDlib/Digital Output  GPIO_Number=GPIO16~GPIO23  GPIO_Bit0=off  GPIO_BIT0_Toggle=off  GPIO_Bit1=off  GPIO_BIT1_Toggle=off  GPIO_Bit2=off  GPIO_BIT2_Toggle=off  GPIO_Bit3=off  GPIO_BIT3_Toggle=off  GPIO_Bit4=off  GPIO_BIT4_Toggle=on  GPIO_Bit5=off  GPIO_BIT5_Toggle=off  GPIO_Bit6=on  GPIO_BIT6_Toggle=off  GPIO_Bit7=off  GPIO_BIT7_Toggle=off
      settings: SourceProductBaseCode=TIC2000
  trigger initialisierung farbe : Subsystem
  gruene_LED : Outport
  n_blau : Outport  Port=2
  n_rot : Outport  Port=3
  wires:
  ADC - Messwerte - Vorverarbeitung (Kennlinien-Steigung und Offset-Kompensation) U_digital = (ADC_in - Offset) * 4.505 V / 4096 mit U_digital_max = 4.505 V U_digital_min = 0 V/1(U_digital) -> Moving Average/1
  Weiche/1(pos) -> Sortierscheibe/5(pos)
  Sortierscheibe/2(n_rot) -> Rate Transition2/1
  Input Farbsensor/1 -> ADC - Messwerte - Vorverarbeitung (Kennlinien-Steigung und Offset-Kompensation) U_digital = (ADC_in - Offset) * 4.505 V / 4096 mit U_digital_max = 4.505 V U_digital_min = 0 V/1(A_IN)
  Entscheidungen je nach Block/5(blau) -> Sortierscheibe/4(blau), Weiche/2(blau)
  Input Fototransistor/1 -> Weiche/1(Block_angekommen), Sortierscheibe/2(Block_angekommen)
  Constant3/1 -> digital out Lichtquelle/1
  Moving Average/1 -> Rate Transition/1
  In2/1 -> Weiche/5(In4)
  Entscheidungen je nach Block/3(rot) -> Weiche/3(rot)
  Sortierscheibe/1(n_blau) -> Rate Transition1/1
  In1/1 -> Sortierscheibe/1(In1)
  Sortierscheibe/5(duty) -> Weiche/6(duty)
  Sortierscheibe/4(schwarz) -> Weiche/7(schwarz_auslenkung)
  Sortierscheibe/3(rot) -> Weiche/8(rot_auslenkung)
  Entscheidungen je nach Block/4(schwarz) -> Weiche/4(schwarz)
  Rate Transition1/1 -> n_blau/1
  Rate Transition2/1 -> n_rot/1
  bereit/1 -> Entscheidungen je nach Block/5(bereit)
  Entscheidungen je nach Block/2(led_rot) -> digital out rote LED/1
  trigger initialisierung farbe/1(trigger1) -> Entscheidungen je nach Block/2(trigger1)
  trigger initialisierung farbe/2(trigger2) -> Entscheidungen je nach Block/3(trigger3)
  trigger initialisierung farbe/3(trigger3) -> Entscheidungen je nach Block/4(trigger2)
  Entscheidungen je nach Block/6(init_farbe) -> Sortierscheibe/3(init_farbe)
  Entscheidungen je nach Block/1(led_gruen) -> gruene_LED/1
  Rate Transition/1 -> Entscheidungen je nach Block/6(U_digital)
  fertig_sortiert/1 -> Entscheidungen je nach Block/1(fertig_sortiert)

== system Gesamtsystem_Prototyp25_01_3/Datenuebertragung zu stehendem System/Berechnung Zustand ==
  In1 : Inport
  In2 : Inport  Port=2
  Switch : Switch  Criteria=u2 > Threshold
  Switch1 : Switch  Criteria=u2 > Threshold  Threshold=1
  Zustand : Constant  OutDataTypeStr=uint16
  Zustand1 : Constant  Value=0  OutDataTypeStr=uint16
  zustand : Outport
  wires:
  In2/1 -> Switch1/2, Switch1/1
  Zustand1/1 -> Switch/3
  Switch/1 -> Switch1/3
  Switch1/1 -> zustand/1
  In1/1 -> Switch/2
  Zustand/1 -> Switch/1

== system Gesamtsystem_Prototyp25_01_3/Kommunikation/I2C Receiver ==
  Trigger : TriggerPort  TriggerType=function-call  VariantControl=(inherit)
  Datastream to bytestream : Subsystem
  Decode Header : Subsystem
  DecodeData : Subsystem  TreatAsAtomicUnit=on
  DecodeNexonar : Subsystem  TreatAsAtomicUnit=on
  I2C Receive1 : c280xlib/I2C Receive  selectModule=I2C_A  addrFormat=7-Bit addressing  saSource=Specify via dialog  SAR=80  bitCount=8  dataLength=14  initValue=0  NACK=on  STP=off  STR=on  sampleTime=-1  dataType=uint16
      settings: SourceProductBaseCode=TIC2000
  I2CFFRX Read : idelinklib_common/Memory Copy  copyFrom=Specified address  copyFromAddressSource=Specify via dialog  copyFromAddress=hex2dec('7321')  copyFromSrcCode=myVariableSrc  dataTypeFrom=uint16  dataDimensionFrom=1  useOffsetFrom=off  offsetFromSrc=Specify via dialog  offsetFrom=0  strideFrom=1  copyTo=Output port  copyToAddressSource=Specify via dialog  copyToAddress=hex2dec('00002000')  copyToSrcCode=myVariableDst  dataTypeTo=uint16  useOffsetTo=off  offsetToSrc=Specify via dialog  offsetTo=0  strideTo=1  sampleTime=-1  useInitValue=off  initValueSrc=Specify constant value  initValue=1  initValueSrcCode=myInitValueVariable  useAsMask=off  maskOperator=bitwise AND  useTermValue=off  termValue=1  isRealtimeEnabled=off  emitCCBeforeWrite=off  CCBeforeWrite=/* Custom Code Before Write*/  emitCCAfterWrite=off  CCAfterWrite=/* Custom Code After Write*/  useDMACopy=off  enableBlockingMode=off
      settings: SourceProductBaseCode=ME
  I2CFFRX Write : idelinklib_common/Memory Copy  copyFrom=Input port  copyFromAddressSource=Input port  copyFromAddress=hex2dec('00001000')  copyFromSrcCode=myVariableSrc  dataTypeFrom=uint16  dataDimensionFrom=1  useOffsetFrom=off  offsetFromSrc=Specify via dialog  offsetFrom=0  strideFrom=1  copyTo=Specified address  copyToAddressSource=Specify via dialog  copyToAddress=hex2dec('7321')  copyToSrcCode=myVariableDst  dataTypeTo=uint16  useOffsetTo=off  offsetToSrc=Specify via dialog  offsetTo=0  strideTo=1  sampleTime=inf  useInitValue=off  initValueSrc=Specify constant value  initValue=1  initValueSrcCode=myInitValueVariable  useAsMask=off  maskOperator=bitwise AND  useTermValue=off  termValue=1  isRealtimeEnabled=off  emitCCBeforeWrite=off  CCBeforeWrite=/* Custom Code Before Write*/  emitCCAfterWrite=off  CCAfterWrite=/* Custom Code After Write*/  useDMACopy=off  enableBlockingMode=off
      settings: SourceProductBaseCode=ME
  RXFFINTCLR : simulink/Logic and Bit Operations/Bit Set  iBit=6
      settings: SourceProductBaseCode=SL
  Terminator : Terminator
  Nexonar (x,y,a,z) : Outport  VectorParamsAs1DForOutWhenUnconnected=off
  Data (8xByte) : Outport  Port=2  VectorParamsAs1DForOutWhenUnconnected=off
  wires:
  I2C Receive1/2 -> Terminator/1
  I2C Receive1/1 -> Datastream to bytestream/1(Datastream)  "I2C_Output_Read"
  Datastream to bytestream/1(Bytes) -> Decode Header/1(Stream), DecodeData/1(Stream), DecodeNexonar/1(Stream)
  Decode Header/2(IsData) -> DecodeData/Enable
  DecodeData/1(Data) -> Data (8xByte)/1
  DecodeNexonar/1(Nexonar) -> Nexonar (x,y,a,z)/1
  Decode Header/1(IsNexonar) -> DecodeNexonar/Enable
  RXFFINTCLR/1 -> I2CFFRX Write/1
  I2CFFRX Read/1 -> RXFFINTCLR/1

== system Gesamtsystem_Prototyp25_01_3/Kommunikation/I2C Reset (behebt Stabilitätsprobleme der I2C-Verbindung) ==
  In1 : Inport
  Constant : Constant  Value=0
  I2C Reinitialisierung : Subsystem  TreatAsAtomicUnit=on
  I2C Reset : Subsystem  TreatAsAtomicUnit=on
  Pulse Generator : DiscretePulseGenerator  Period=50  SampleTime=0.001
  Switch : Switch  Criteria=u2 > Threshold
  wires:
  Switch/1 -> I2C Reset/Trigger, I2C Reinitialisierung/Trigger
  Constant/1 -> Switch/1
  Pulse Generator/1 -> Switch/3
  In1/1 -> Switch/2

== system Gesamtsystem_Prototyp25_01_3/Kommunikation/I2C Transmitter ==
  In1 : Inport
  Trigger : TriggerPort  VariantControl=Variant  PortDimensions=1
  Receive1 : Receive  InputPortMessageModes=m  UseInternalQueue=off  QueueOverwriting=on  QueueLength=1  QueueType=LIFO  ShowQueueStatus=on
      settings: OutputPortMap=o0,o1
  Scope : Scope
  Subsystem : Subsystem
  Terminator : Terminator
  wires:
  In1/1 -> Receive1/1
  Subsystem/1(Out1) -> Scope/1, Terminator/1
  Receive1/2 -> Subsystem/1(In1)
  Receive1/1 -> Subsystem/Enable

== system Gesamtsystem_Prototyp25_01_3/Kommunikation/Pack Data Message ==
  Data : Inport
  Trigger : TriggerPort  VariantControl=Variant  PortDimensions=1
  I2C_MARKER_COMMS_DATA_OUT : Constant  Value=hex2dec('0022')  OutDataTypeStr=uint16
  I2C_MSG_END1 : Constant  Value=hex2dec('00D7')  OutDataTypeStr=uint16
  I2C_MSG_END2 : Constant  Value=hex2dec('002E')  OutDataTypeStr=uint16
  I2C_MSG_START1 : Constant  Value=hex2dec('00E2')  OutDataTypeStr=uint16
  I2C_MSG_START2 : Constant  Value=hex2dec('007D')  OutDataTypeStr=uint16
  Mux : Mux  Inputs=8
  Pack Data Bytes : Subsystem
  Pad : dspsigops/Pad  padAlong=Columns  dimsToPad=1  valSrc=Specify via dialog  padVal=255  spec=Output size  padNumOutRowsSpecMethod=User-specified  numOutRows=16  padNumOutColsSpecMethod=User-specified  numOutCols=1  isVarDimsMode=off  padBeginning=0  padEnd=0  outSizeMode=User-specified  outSize=1  padSigAt=End  trunc_flag=None  roundingMode=Floor  overflowMode=off  truncOrWrapMode=Truncate  wrap_flag=None
      settings: SourceProductBaseCode=DS
  Total Length : Constant  Value=14  OutDataTypeStr=uint16
  Message : Outport
  wires:
  Pad/1 -> Message/1
  Mux/1 -> Pad/1
  I2C_MSG_END2/1 -> Mux/8
  I2C_MSG_START2/1 -> Mux/3
  I2C_MSG_END1/1 -> Mux/7
  Total Length/1 -> Mux/5
  I2C_MARKER_COMMS_DATA_OUT/1 -> Mux/4
  I2C_MSG_START1/1 -> Mux/1, Mux/2
  Data/1 -> Pack Data Bytes/1(in)
  Pack Data Bytes/1(out) -> Mux/6

== system Gesamtsystem_Prototyp25_01_3/Kommunikation/Pack Wifi Config Message ==
  Own ID1 : Inport
  Partner ID1 : Inport  Port=2
  Nexonar ID1 : Inport  Port=3
  I2C_MARKER_WIFI_CONFIG : Constant  Value=hex2dec('0005')  OutDataTypeStr=uint16
  I2C_MSG_END1 : Constant  Value=hex2dec('00D7')  OutDataTypeStr=uint16
  I2C_MSG_END2 : Constant  Value=hex2dec('002E')  OutDataTypeStr=uint16
  I2C_MSG_START1 : Constant  Value=hex2dec('00E2')  OutDataTypeStr=uint16
  I2C_MSG_START2 : Constant  Value=hex2dec('007D')  OutDataTypeStr=uint16
  Mux : Mux  Inputs=10
  Pad : dspsigops/Pad  padAlong=Rows  dimsToPad=1  valSrc=Specify via dialog  padVal=255  spec=Output size  padNumOutRowsSpecMethod=User-specified  numOutRows=113-60  padNumOutColsSpecMethod=User-specified  numOutCols=16  isVarDimsMode=off  padBeginning=0  padEnd=0  outSizeMode=User-specified  outSize=1  padSigAt=End  trunc_flag=None  roundingMode=Floor  overflowMode=off  truncOrWrapMode=Truncate  wrap_flag=None
      settings: SourceProductBaseCode=DS
  Total Length : Constant  Value=9  OutDataTypeStr=uint16
  Message : Outport
  wires:
  I2C_MSG_END2/1 -> Mux/10
  I2C_MSG_END1/1 -> Mux/9
  Mux/1 -> Pad/1
  Pad/1 -> Message/1
  I2C_MSG_START1/1 -> Mux/1, Mux/2
  Total Length/1 -> Mux/5
  I2C_MARKER_WIFI_CONFIG/1 -> Mux/4
  I2C_MSG_START2/1 -> Mux/3
  Nexonar ID1/1 -> Mux/8
  Partner ID1/1 -> Mux/7
  Own ID1/1 -> Mux/6

== system Gesamtsystem_Prototyp25_01_3/Kommunikation/Send to Queue ==
  In1 : Inport
  Trigger : TriggerPort  VariantControl=Variant  PortDimensions=1
  Send : Send  OutputPortMessageModes=m
  Out1 : Outport
  wires:
  In1/1 -> Send/1
  Send/1 -> Out1/1

== system Gesamtsystem_Prototyp25_01_3/Kommunikation/Subsystem ==
  In1 : Inport
  Bit Shift : hdlsllib/Logic and Bit Operations/Bit Shift  mode=Shift Left Logical  N=8
  Deinterlacer : commsequence2/Deinterlacer
      settings: SourceProductBaseCode=CM
  Rate Transition : RateTransition  Commented=through
  Sum : Sum  Inputs=|++
  Out1 : Outport
  wires:
  In1/1 -> Deinterlacer/1
  Deinterlacer/2 -> Bit Shift/1
  Deinterlacer/1 -> Sum/1
  Bit Shift/1 -> Sum/2
  Sum/1 -> Rate Transition/1
  Rate Transition/1 -> Out1/1

== system Gesamtsystem_Prototyp25_01_3/Kommunikation/Subsystem1 ==
  In : Inport
  Data Type Conversion : DataTypeConversion  OutDataTypeStr=uint16
  Delay1 : Delay
  Relational Operator : RelationalOperator  Operator=~=  OutDataTypeStr=fixdt(1,16)  RndMeth=Simplest
  Change : Outport
  wires:
  In/1 -> Delay1/1, Relational Operator/1
  Relational Operator/1 -> Data Type Conversion/1
  Data Type Conversion/1 -> Change/1
  Delay1/1 -> Relational Operator/2

== system Gesamtsystem_Prototyp25_01_3/Kommunikation/Subsystem2 ==
  In : Inport
  Data Type Conversion : DataTypeConversion  OutDataTypeStr=uint16
  Delay1 : Delay
  Relational Operator : RelationalOperator  Operator=~=  OutDataTypeStr=fixdt(1,16)  RndMeth=Simplest
  Change : Outport
  wires:
  Delay1/1 -> Relational Operator/2
  Data Type Conversion/1 -> Change/1
  Relational Operator/1 -> Data Type Conversion/1
  In/1 -> Relational Operator/1, Delay1/1

== system Gesamtsystem_Prototyp25_01_3/Motor Module Lampe Aufzug Ruettler/Inverter ==
  ende : Inport
  Constant2 : Constant  Value=0
  Constant3 : Constant
  Switch : Switch  Criteria=u2 > Threshold  Threshold=0.5
  ende_nicht : Outport
  wires:
  Constant2/1 -> Switch/1
  Constant3/1 -> Switch/3
  ende/1 -> Switch/2
  Switch/1 -> ende_nicht/1

== system Gesamtsystem_Prototyp25_01_3/Navigation und Uebergabe/Abwurf und Uebergabe ==
  rb : Inport
  s : Inport  Port=2
  rb_dir : Inport  Port=3
  Abgabe_S_R_B : Stateflow chart  TreatAsAtomicUnit=on
      settings: PortSchema="{\"entries\":[{\"content\":{\"sides\":[{\"content\":{\"connectorIds\":[\"In1\",\"In2\",\"In3\"]},\"type\":\"ConnectorPlacement.EquallySpacedRectSide\",\"uuid\":\"6b94dce2-58bc-4163-84c5-0ea74a97faba\"},{\"content\":{\"connectorIds\":[\"Out1\",\"Out3\",\"Out4\",\"Out2\"],\"side\":\"RIGHT\"},\"type\":\"ConnectorPlacement.EquallySpacedRectSide\",\"uuid\":\"bf0e1c86-98a0-46d4-9bfe-90681bf0c414\"},{\"content\":{\"connectorIds\":[],\"side\":\"TOP\"},\"type\":\"ConnectorPlacement.EquallySpacedRectSide\",\"uuid\":\"c6fc9323-e37d-4199-b015-4c2902c4c741\"}]},\"type\":\"ConnectorPlacement.EquallySpacedConnector\",\"uuid\":\"dfe069ec-4002-4cf5-9b97-633b6ee58dee\"}],\"packageUris\":[\"http://schema.mathworks.com/mf0/Connector/R2020b\"],\"version\":\"1.0\"}"
  Drehrichtungsvorgabe Abwurf : c2837xDlib/Digital Output  GPIO_Number=GPIO24~GPIO31  GPIO_Bit0=off  GPIO_BIT0_Toggle=off  GPIO_Bit1=off  GPIO_BIT1_Toggle=off  GPIO_Bit2=on  GPIO_BIT2_Toggle=off  GPIO_Bit3=off  GPIO_BIT3_Toggle=off  GPIO_Bit4=off  GPIO_BIT4_Toggle=off  GPIO_Bit5=off  GPIO_BIT5_Toggle=off  GPIO_Bit6=off  GPIO_BIT6_Toggle=off  GPIO_Bit7=off  GPIO_BIT7_Toggle=off
      settings: SourceProductBaseCode=TIC2000
  Drehrichtungsvorgabe Uebergabe : c2837xDlib/Digital Output  GPIO_Number=GPIO24~GPIO31  GPIO_Bit0=off  GPIO_BIT0_Toggle=off  GPIO_Bit1=off  GPIO_BIT1_Toggle=off  GPIO_Bit2=off  GPIO_BIT2_Toggle=off  GPIO_Bit3=on  GPIO_BIT3_Toggle=off  GPIO_Bit4=off  GPIO_BIT4_Toggle=off  GPIO_Bit5=off  GPIO_BIT5_Toggle=off  GPIO_Bit6=off  GPIO_BIT6_Toggle=off  GPIO_Bit7=off  GPIO_BIT7_Toggle=off
      settings: SourceProductBaseCode=TIC2000
  "P-Regler mit Regelfehler Begrenzung Initial: k = 0.1, limit = +/- 100 Sampletime 0.1" : Subsystem
  "P-Regler mit Regelfehler Begrenzung Initial: k = 0.1, limit = +/- 100 Sampletime 0.2" : Subsystem
  PWM Uebergabe : Outport
  PWM Abwurf : Outport  Port=2
  wires:
  Abgabe_S_R_B/3(y_ist_rb) -> "P-Regler mit Regelfehler Begrenzung Initial: k = 0.1, limit = +/- 100 Sampletime 0.1"/2(y_ist)
  rb/1 -> Abgabe_S_R_B/1(rb)
  Abgabe_S_R_B/4(y_soll_s) -> "P-Regler mit Regelfehler Begrenzung Initial: k = 0.1, limit = +/- 100 Sampletime 0.2"/1(y_soll_s)
  Abgabe_S_R_B/1(y_soll_rb) -> "P-Regler mit Regelfehler Begrenzung Initial: k = 0.1, limit = +/- 100 Sampletime 0.1"/1(y_soll_rb)
  "P-Regler mit Regelfehler Begrenzung Initial: k = 0.1, limit = +/- 100 Sampletime 0.2"/2(r/l_out) -> Drehrichtungsvorgabe Abwurf/1
  "P-Regler mit Regelfehler Begrenzung Initial: k = 0.1, limit = +/- 100 Sampletime 0.2"/1(pwm_out) -> PWM Abwurf/1
  "P-Regler mit Regelfehler Begrenzung Initial: k = 0.1, limit = +/- 100 Sampletime 0.1"/2(r/l_out) -> Drehrichtungsvorgabe Uebergabe/1
  "P-Regler mit Regelfehler Begrenzung Initial: k = 0.1, limit = +/- 100 Sampletime 0.1"/1(pwm_out) -> PWM Uebergabe/1
  s/1 -> Abgabe_S_R_B/2(s)
  rb_dir/1 -> Abgabe_S_R_B/3(rb_dir)
  Abgabe_S_R_B/2(y_ist_s) -> "P-Regler mit Regelfehler Begrenzung Initial: k = 0.1, limit = +/- 100 Sampletime 0.2"/2(y_ist)

== system Gesamtsystem_Prototyp25_01_3/Navigation und Uebergabe/Eingabeschalter Positionen ==
  Digital Input : c2837xDlib/Digital Input  GPIO_Number=GPIO16~GPIO23  GPIO_Bit0=on  GPIO_Bit1=off  GPIO_Bit2=off  GPIO_Bit3=off  GPIO_Bit4=off  GPIO_Bit5=off  GPIO_Bit6=off  GPIO_Bit7=off  sampleTime=0.1  dataType=auto  GPIO_Bit0_Qualification=Sync to SYSCLKOUT  GPIO_Bit1_Qualification=Sync to SYSCLKOUT  GPIO_Bit2_Qualification=Sync to SYSCLKOUT  GPIO_Bit3_Qualification=Sync to SYSCLKOUT  GPIO_Bit4_Qualification=Sync to SYSCLKOUT  GPIO_Bit5_Qualification=Sync to SYSCLKOUT  GPIO_Bit6_Qualification=Sync to SYSCLKOUT  GPIO_Bit7_Qualification=Sync to SYSCLKOUT  Qualification_Period=-1
      settings: SourceProductBaseCode=TIC2000
  Digital Input1 : c2837xDlib/Digital Input  GPIO_Number=GPIO120~GPIO127  GPIO_Bit0=off  GPIO_Bit1=off  GPIO_Bit2=off  GPIO_Bit3=off  GPIO_Bit4=on  GPIO_Bit5=off  GPIO_Bit6=off  GPIO_Bit7=off  sampleTime=0.1  dataType=auto  GPIO_Bit0_Qualification=Sync to SYSCLKOUT  GPIO_Bit1_Qualification=Sync to SYSCLKOUT  GPIO_Bit2_Qualification=Sync to SYSCLKOUT  GPIO_Bit3_Qualification=Sync to SYSCLKOUT  GPIO_Bit4_Qualification=Sync to SYSCLKOUT  GPIO_Bit5_Qualification=Sync to SYSCLKOUT  GPIO_Bit6_Qualification=Sync to SYSCLKOUT  GPIO_Bit7_Qualification=Sync to SYSCLKOUT  Qualification_Period=-1
      settings: SourceProductBaseCode=TIC2000
  Logical Operator : Logic  Operator=OR  AllPortsSameDT=off  OutDataTypeStr=boolean
  trigger : Outport
  wires:
  Logical Operator/1 -> trigger/1
  Digital Input/1 -> Logical Operator/1
  Digital Input1/1 -> Logical Operator/2

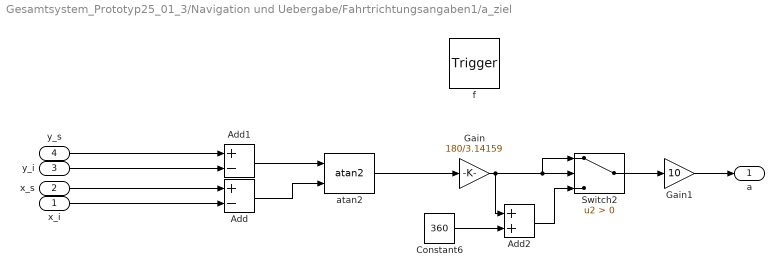
== system Gesamtsystem_Prototyp25_01_3/Navigation und Uebergabe/Fahrtrichtungsangaben1/a_ziel ==
  x_i : Inport  OutDataTypeStr=double  PortDimensions=1
  x_s : Inport  Port=2  OutDataTypeStr=double  PortDimensions=1
  y_i : Inport  Port=3  OutDataTypeStr=double  PortDimensions=1
  y_s : Inport  Port=4  OutDataTypeStr=double  PortDimensions=1
  f : TriggerPort  TriggerType=function-call  VariantControl=(inherit)
      settings: CopyFcn=Stateflow.SLINSF.SimulinkMan.removeBlockPreDeleteFcn  PreDeleteFcn=Stateflow.SLINSF.SimulinkMan.unsafePredeleteFcn
  Add : Sum  Inputs=+-
  Add1 : Sum  Inputs=+-
  Add2 : Sum
  Constant6 : Constant  Value=360
  Gain : Gain  Gain=180/3.14159
  Gain1 : Gain  Gain=10  ParamDataTypeStr=uint16  OutDataTypeStr=double
  Switch2 : Switch  Criteria=u2 > Threshold
  atan2 : mcbcontrolslib/atan2  outputUnit=Radians
      settings: SourceProductBaseCode=MT
  a : Outport  OutDataTypeStr=double
  wires:
  Gain1/1 -> a/1
  Add/1 -> atan2/2
  Switch2/1 -> Gain1/1
  Add1/1 -> atan2/1
  Gain/1 -> Add2/1, Switch2/1, Switch2/2
  atan2/1 -> Gain/1
  Constant6/1 -> Add2/2
  Add2/1 -> Switch2/3
  y_s/1 -> Add1/1
  y_i/1 -> Add1/2
  x_s/1 -> Add/1
  x_i/1 -> Add/2

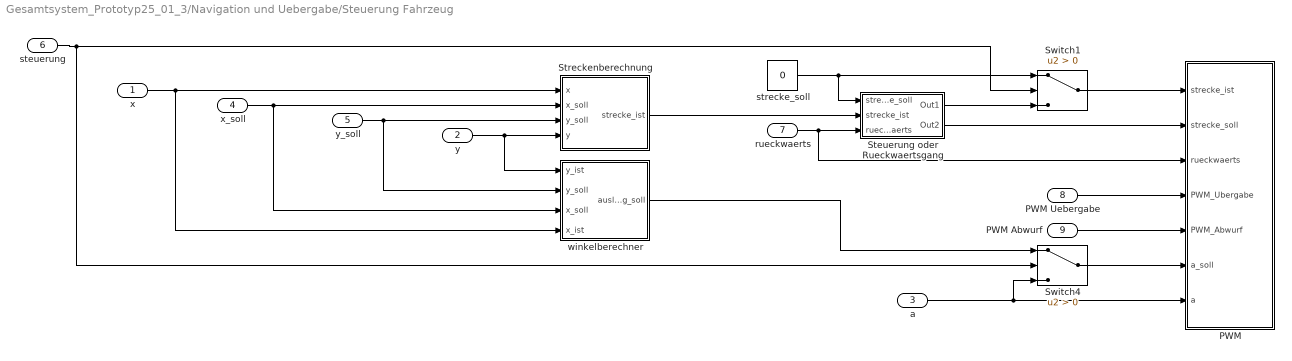
== system Gesamtsystem_Prototyp25_01_3/Navigation und Uebergabe/Steuerung Fahrzeug ==
  x : Inport
  y : Inport  Port=2
  a : Inport  Port=3
  x_soll : Inport  Port=4
  y_soll : Inport  Port=5
  steuerung : Inport  Port=6
  rueckwaerts : Inport  Port=7
  PWM Uebergabe : Inport  Port=8
  PWM Abwurf : Inport  Port=9
  PWM : Subsystem
  Steuerung oder Rueckwaertsgang : Subsystem
  Streckenberechnung : Subsystem
  Switch1 : Switch  Criteria=u2 > Threshold
  Switch4 : Switch  Criteria=u2 > Threshold
  strecke_soll : Constant  Value=0
  winkelberechner : Subsystem
  wires:
  Steuerung oder Rueckwaertsgang/2(Out2) -> PWM/2(strecke_soll)
  steuerung/1 -> Switch4/2, Switch1/2
  Steuerung oder Rueckwaertsgang/1(Out1) -> Switch1/3
  rueckwaerts/1 -> Steuerung oder Rueckwaertsgang/3(rueckwaerts), PWM/3(rueckwaerts)
  y_soll/1 -> winkelberechner/2(y_soll), Streckenberechnung/3(y_soll)
  winkelberechner/1(auslenkung_soll) -> Switch4/1
  strecke_soll/1 -> Steuerung oder Rueckwaertsgang/1(strecke_soll), Switch1/1
  Switch4/1 -> PWM/6(a_soll)
  y/1 -> winkelberechner/1(y_ist), Streckenberechnung/4(y)
  x_soll/1 -> winkelberechner/3(x_soll), Streckenberechnung/2(x_soll)
  x/1 -> Streckenberechnung/1(x), winkelberechner/4(x_ist)
  a/1 -> Switch4/3, PWM/7(a)
  Streckenberechnung/1(strecke_ist) -> Steuerung oder Rueckwaertsgang/2(strecke_ist)
  PWM Uebergabe/1 -> PWM/4(PWM_Ubergabe)
  Switch1/1 -> PWM/1(strecke_ist)
  PWM Abwurf/1 -> PWM/5(PWM_Abwurf)

== system Gesamtsystem_Prototyp25_01_3/Navigation und Uebergabe/Trigger Andock ==
  Digital Input1 : c2837xDlib/Digital Input  GPIO_Number=GPIO24~GPIO31  GPIO_Bit0=on  GPIO_Bit1=off  GPIO_Bit2=off  GPIO_Bit3=off  GPIO_Bit4=off  GPIO_Bit5=off  GPIO_Bit6=off  GPIO_Bit7=off  sampleTime=1  dataType=auto  GPIO_Bit0_Qualification=Sync to SYSCLKOUT  GPIO_Bit1_Qualification=Sync to SYSCLKOUT  GPIO_Bit2_Qualification=Sync to SYSCLKOUT  GPIO_Bit3_Qualification=Sync to SYSCLKOUT  GPIO_Bit4_Qualification=Sync to SYSCLKOUT  GPIO_Bit5_Qualification=Sync to SYSCLKOUT  GPIO_Bit6_Qualification=Sync to SYSCLKOUT  GPIO_Bit7_Qualification=Sync to SYSCLKOUT  Qualification_Period=-1
      settings: SourceProductBaseCode=TIC2000
  Digital Input2 : c2837xDlib/Digital Input  GPIO_Number=GPIO0~GPIO7  GPIO_Bit0=off  GPIO_Bit1=off  GPIO_Bit2=off  GPIO_Bit3=off  GPIO_Bit4=off  GPIO_Bit5=on  GPIO_Bit6=off  GPIO_Bit7=off  sampleTime=1  dataType=auto  GPIO_Bit0_Qualification=Sync to SYSCLKOUT  GPIO_Bit1_Qualification=Sync to SYSCLKOUT  GPIO_Bit2_Qualification=Sync to SYSCLKOUT  GPIO_Bit3_Qualification=Sync to SYSCLKOUT  GPIO_Bit4_Qualification=Sync to SYSCLKOUT  GPIO_Bit5_Qualification=Sync to SYSCLKOUT  GPIO_Bit6_Qualification=Sync to SYSCLKOUT  GPIO_Bit7_Qualification=Sync to SYSCLKOUT  Qualification_Period=-1
      settings: SourceProductBaseCode=TIC2000
  Logical Operator : Logic  Operator=OR  AllPortsSameDT=off  OutDataTypeStr=boolean
  andock_l : Outport  OutDataTypeStr=boolean
  andock_r : Outport  Port=2  OutDataTypeStr=boolean
  andock : Outport  Port=3  OutDataTypeStr=boolean
  wires:
  Digital Input2/1 -> andock_l/1, Logical Operator/1
  Digital Input1/1 -> Logical Operator/2, andock_r/1
  Logical Operator/1 -> andock/1

== system Gesamtsystem_Prototyp25_01_3/Sortierung/ADC - Messwerte - Vorverarbeitung (Kennlinien-Steigung und Offset-Kompensation) U_digital = (ADC_in - Offset) * 4.505 V // 4096 mit U_digital_max = 4.505 V U_digital_min = 0 V ==
  A_IN : Inport
  Add : Sum
  Offset : Constant  Value=0
  Verstaerkung : Gain  Gain=4.505/4096
  U_digital : Outport  VectorParamsAs1DForOutWhenUnconnected=off
  wires:
  Verstaerkung/1 -> U_digital/1
  Add/1 -> Verstaerkung/1
  A_IN/1 -> Add/2
  Offset/1 -> Add/1
